simulink model "TractionControl"  (R2024b)
settings: configuration reference "STM32H7_Config" (kept outside this file)
undefined symbols (not defined in the file): Ki1, MMotorMinAllowed, rStraightSlipRatio
libraries: simulink x2
settings Model: DataDictionary=Master_Dictionary.sldd  EnableAccessToBaseWorkspace=off  Creator=torni  LastModifiedBy=William
settings ConfigSetRef: SourceName=STM32H7_Config

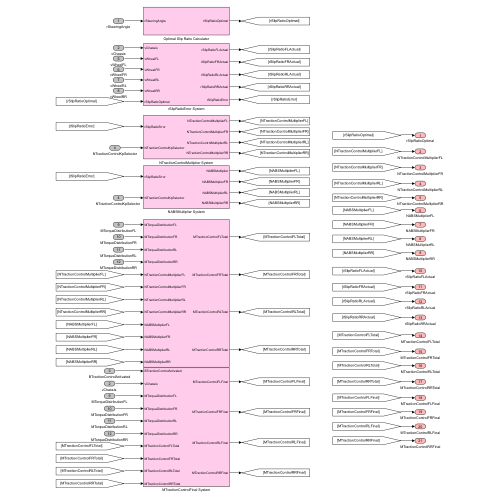
[thumbnail: Simulink's stored preview of the top-level diagram]
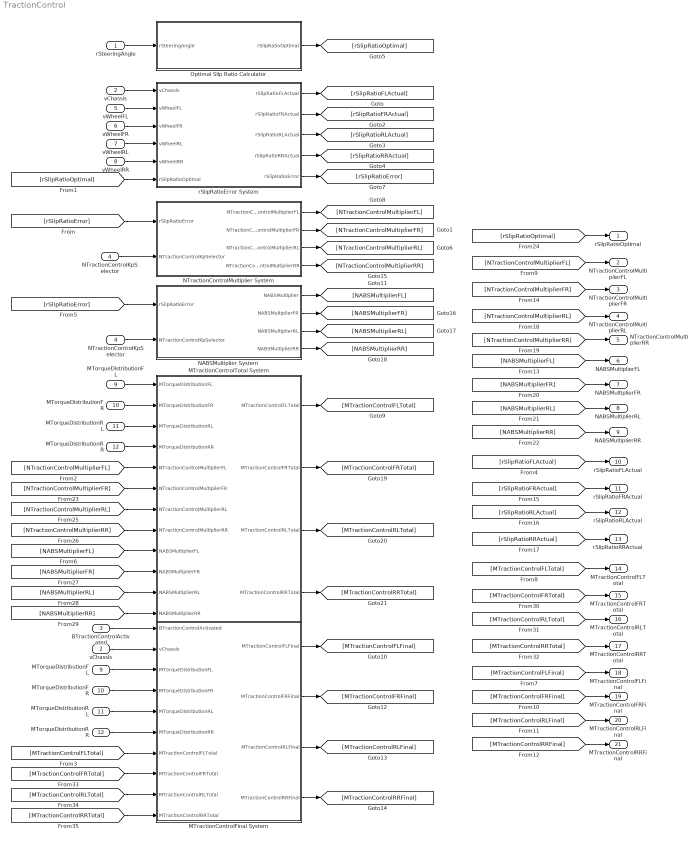
== system TractionControl ==
  rSteeringAngle : Inport  OutDataTypeStr=double
  vChassis : Inport  Port=2  OutDataTypeStr=double
  BTractionControlActivated : Inport  Port=3  OutDataTypeStr=boolean
  NTractionControlKpSelector : Inport  Port=4  OutDataTypeStr=double
  vWheelFL : Inport  Port=5  OutDataTypeStr=double  LockScale=on
  vWheelFR : Inport  Port=6  OutDataTypeStr=double  LockScale=on
  vWheelRL : Inport  Port=7  OutDataTypeStr=double  LockScale=on
  vWheelRR : Inport  Port=8  OutDataTypeStr=double  LockScale=on
  MTorqueDistributionFL : Inport  Port=9  OutDataTypeStr=double
  MTorqueDistributionFR : Inport  Port=10  OutDataTypeStr=double
  MTorqueDistributionRL : Inport  Port=11  OutDataTypeStr=double
  MTorqueDistributionRR : Inport  Port=12  OutDataTypeStr=double
  "MTorqueDistributionFL " : InportShadow  Port=9  OutDataTypeStr=double
  "MTorqueDistributionFR " : InportShadow  Port=10  OutDataTypeStr=double
  "MTorqueDistributionRL " : InportShadow  Port=11  OutDataTypeStr=double
  "MTorqueDistributionRR " : InportShadow  Port=12  OutDataTypeStr=double
  MTractionControlFinal System : Subsystem
  MTractionControlTotal System : Subsystem
  NABSMultiplier System : Subsystem
  "NTractionControlKpSelector " : InportShadow  Port=4  OutDataTypeStr=double
  NTractionControlMultiplier System : Subsystem
  Optimal Slip Ratio Calculator : Subsystem
  rSlipRatioError System : Subsystem
  "vChassis " : InportShadow  Port=2  OutDataTypeStr=double
  rSlipRatioOptimal : Outport  OutDataTypeStr=double  VectorParamsAs1DForOutWhenUnconnected=off
  NTractionControlMultiplierFL : Outport  Port=2  OutDataTypeStr=double  VectorParamsAs1DForOutWhenUnconnected=off
  NTractionControlMultiplierFR : Outport  Port=3  OutDataTypeStr=double  VectorParamsAs1DForOutWhenUnconnected=off
  NTractionControlMultiplierRL : Outport  Port=4  OutDataTypeStr=double  VectorParamsAs1DForOutWhenUnconnected=off
  NTractionControlMultiplierRR : Outport  Port=5  OutDataTypeStr=double  VectorParamsAs1DForOutWhenUnconnected=off
  NABSMultiplierFL : Outport  Port=6  OutDataTypeStr=double  VectorParamsAs1DForOutWhenUnconnected=off
  NABSMultiplierFR : Outport  Port=7  OutDataTypeStr=double  VectorParamsAs1DForOutWhenUnconnected=off
  NABSMultiplierRL : Outport  Port=8  OutDataTypeStr=double  VectorParamsAs1DForOutWhenUnconnected=off
  NABSMultiplierRR : Outport  Port=9  OutDataTypeStr=double  VectorParamsAs1DForOutWhenUnconnected=off
  rSlipRatioFLActual : Outport  Port=10  OutDataTypeStr=double  VectorParamsAs1DForOutWhenUnconnected=off
  rSlipRatioFRActual : Outport  Port=11  OutDataTypeStr=double  VectorParamsAs1DForOutWhenUnconnected=off
  rSlipRatioRLActual : Outport  Port=12  OutDataTypeStr=double  VectorParamsAs1DForOutWhenUnconnected=off
  rSlipRatioRRActual : Outport  Port=13  OutDataTypeStr=double  VectorParamsAs1DForOutWhenUnconnected=off
  MTractionControlFLTotal : Outport  Port=14  OutDataTypeStr=double  VectorParamsAs1DForOutWhenUnconnected=off
  MTractionControlFRTotal : Outport  Port=15  OutDataTypeStr=double  VectorParamsAs1DForOutWhenUnconnected=off
  MTractionControlRLTotal : Outport  Port=16  OutDataTypeStr=double  VectorParamsAs1DForOutWhenUnconnected=off
  MTractionControlRRTotal : Outport  Port=17  OutDataTypeStr=double  VectorParamsAs1DForOutWhenUnconnected=off
  MTractionControlFLFinal : Outport  Port=18  OutDataTypeStr=double  VectorParamsAs1DForOutWhenUnconnected=off
  MTractionControlFRFinal : Outport  Port=19  OutDataTypeStr=double  VectorParamsAs1DForOutWhenUnconnected=off
  MTractionControlRLFinal : Outport  Port=20  OutDataTypeStr=double  VectorParamsAs1DForOutWhenUnconnected=off
  MTractionControlRRFinal : Outport  Port=21  OutDataTypeStr=double  VectorParamsAs1DForOutWhenUnconnected=off
  wires:
  rSteeringAngle/1 -> Optimal Slip Ratio Calculator/1(rSteeringAngle)
  Optimal Slip Ratio Calculator/1(rSlipRatioOptimal) -> [rSlipRatioOptimal]
  [rSlipRatioOptimal] -> rSlipRatioOptimal/1
  MTorqueDistributionFL/1 -> MTractionControlTotal System/1(MTorqueDistributionFL)
  MTorqueDistributionFR/1 -> MTractionControlTotal System/2(MTorqueDistributionFR)
  vWheelRR/1 -> rSlipRatioError System/5(vWheelRR)
  NABSMultiplier System/1(NABSMultiplier) -> [NABSMultiplierFL]
  [rSlipRatioError] -> NTractionControlMultiplier System/1(rSlipRatioError)
  NTractionControlMultiplier System/1(NTractionControlMultiplierFL) -> [NTractionControlMultiplierFL]
  vChassis/1 -> rSlipRatioError System/1(vChassis)
  vWheelFL/1 -> rSlipRatioError System/2(vWheelFL)
  "vChassis "/1 -> MTractionControlFinal System/2(vChassis)
  vWheelFR/1 -> rSlipRatioError System/3(vWheelFR)
  [NTractionControlMultiplierFL] -> NTractionControlMultiplierFL/1
  MTractionControlTotal System/1(MTractionControlFLTotal) -> [MTractionControlFLTotal]
  "MTorqueDistributionFL "/1 -> MTractionControlFinal System/3(MTorqueDistributionFL)
  "NTractionControlKpSelector "/1 -> NABSMultiplier System/2(NTractionControlKpSelector)
  [rSlipRatioError] -> NABSMultiplier System/1(rSlipRatioError)
  "MTorqueDistributionRR "/1 -> MTractionControlFinal System/6(MTorqueDistributionRR)
  BTractionControlActivated/1 -> MTractionControlFinal System/1(BTractionControlActivated)
  "MTorqueDistributionRL "/1 -> MTractionControlFinal System/5(MTorqueDistributionRL)
  [NABSMultiplierFL] -> MTractionControlTotal System/9(NABSMultiplierFL)
  MTorqueDistributionRL/1 -> MTractionControlTotal System/3(MTorqueDistributionRL)
  "MTorqueDistributionFR "/1 -> MTractionControlFinal System/4(MTorqueDistributionFR)
  [NTractionControlMultiplierFL] -> MTractionControlTotal System/5(NTractionControlMultiplierFL)
  MTractionControlFinal System/1(MTractionControlFLFinal) -> [MTractionControlFLFinal]
  rSlipRatioError System/1(rSlipRatioFLActual) -> [rSlipRatioFLActual]
  vWheelRL/1 -> rSlipRatioError System/4(vWheelRL)
  MTractionControlFinal System/3(MTractionControlRLFinal) -> [MTractionControlRLFinal]
  MTractionControlFinal System/4(MTractionControlRRFinal) -> [MTractionControlRRFinal]
  MTractionControlFinal System/2(MTractionControlFRFinal) -> [MTractionControlFRFinal]
  NTractionControlKpSelector/1 -> NTractionControlMultiplier System/2(NTractionControlKpSelector)
  MTorqueDistributionRR/1 -> MTractionControlTotal System/4(MTorqueDistributionRR)
  [rSlipRatioOptimal] -> rSlipRatioError System/6(rSlipRatioOptimal)
  rSlipRatioError System/5(rSlipRatioError) -> [rSlipRatioError]
  rSlipRatioError System/2(rSlipRatioFRActual) -> [rSlipRatioFRActual]
  rSlipRatioError System/3(rSlipRatioRLActual) -> [rSlipRatioRLActual]
  rSlipRatioError System/4(rSlipRatioRRActual) -> [rSlipRatioRRActual]
  NTractionControlMultiplier System/2(NTractionControlMultiplierFR) -> [NTractionControlMultiplierFR]
  NTractionControlMultiplier System/3(NTractionControlMultiplierRL) -> [NTractionControlMultiplierRL]
  NTractionControlMultiplier System/4(NTractionControlMultiplierRR) -> [NTractionControlMultiplierRR]
  [NTractionControlMultiplierFR] -> NTractionControlMultiplierFR/1
  [NTractionControlMultiplierRL] -> NTractionControlMultiplierRL/1
  [NTractionControlMultiplierRR] -> NTractionControlMultiplierRR/1
  [NABSMultiplierFL] -> NABSMultiplierFL/1
  NABSMultiplier System/4(NABSMultiplierRR) -> [NABSMultiplierRR]
  NABSMultiplier System/3(NABSMultiplierRL) -> [NABSMultiplierRL]
  NABSMultiplier System/2(NABSMultiplierFR) -> [NABSMultiplierFR]
  [NTractionControlMultiplierFR] -> MTractionControlTotal System/6(NTractionControlMultiplierFR)
  [NTractionControlMultiplierRL] -> MTractionControlTotal System/7(NTractionControlMultiplierRL)
  [NTractionControlMultiplierRR] -> MTractionControlTotal System/8(NTractionControlMultiplierRR)
  [NABSMultiplierRR] -> NABSMultiplierRR/1
  [NABSMultiplierRL] -> NABSMultiplierRL/1
  [NABSMultiplierFR] -> NABSMultiplierFR/1
  [NABSMultiplierFR] -> MTractionControlTotal System/10(NABSMultiplierFR)
  [NABSMultiplierRL] -> MTractionControlTotal System/11(NABSMultiplierRL)
  [NABSMultiplierRR] -> MTractionControlTotal System/12(NABSMultiplierRR)
  [rSlipRatioRRActual] -> rSlipRatioRRActual/1
  [rSlipRatioFLActual] -> rSlipRatioFLActual/1
  [rSlipRatioFRActual] -> rSlipRatioFRActual/1
  [rSlipRatioRLActual] -> rSlipRatioRLActual/1
  MTractionControlTotal System/2(MTractionControlFRTotal) -> [MTractionControlFRTotal]
  MTractionControlTotal System/3(MTractionControlRLTotal) -> [MTractionControlRLTotal]
  MTractionControlTotal System/4(MTractionControlRRTotal) -> [MTractionControlRRTotal]
  [MTractionControlFLTotal] -> MTractionControlFLTotal/1
  [MTractionControlFRTotal] -> MTractionControlFRTotal/1
  [MTractionControlRLTotal] -> MTractionControlRLTotal/1
  [MTractionControlRRTotal] -> MTractionControlRRTotal/1
  [MTractionControlFLFinal] -> MTractionControlFLFinal/1
  [MTractionControlRRFinal] -> MTractionControlRRFinal/1
  [MTractionControlFRFinal] -> MTractionControlFRFinal/1
  [MTractionControlRLFinal] -> MTractionControlRLFinal/1
  [MTractionControlFLTotal] -> MTractionControlFinal System/7(MTractionControlFLTotal)
  [MTractionControlFRTotal] -> MTractionControlFinal System/8(MTractionControlFRTotal)
  [MTractionControlRLTotal] -> MTractionControlFinal System/9(MTractionControlRLTotal)
  [MTractionControlRRTotal] -> MTractionControlFinal System/10(MTractionControlRRTotal)

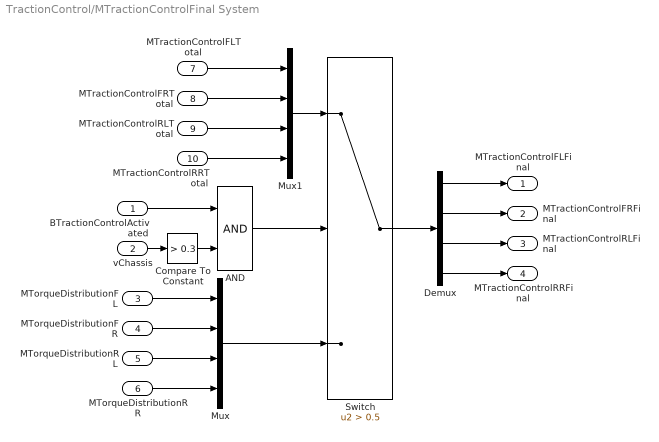
== system TractionControl/MTractionControlFinal System ==
  BTractionControlActivated : Inport  OutDataTypeStr=boolean
  vChassis : Inport  Port=2  OutDataTypeStr=double
  MTorqueDistributionFL : Inport  Port=3  OutDataTypeStr=double
  MTorqueDistributionFR : Inport  Port=4  OutDataTypeStr=double
  MTorqueDistributionRL : Inport  Port=5  OutDataTypeStr=double
  MTorqueDistributionRR : Inport  Port=6  OutDataTypeStr=double
  MTractionControlFLTotal : Inport  Port=7  OutDataTypeStr=double
  MTractionControlFRTotal : Inport  Port=8  OutDataTypeStr=double
  MTractionControlRLTotal : Inport  Port=9  OutDataTypeStr=double
  MTractionControlRRTotal : Inport  Port=10  OutDataTypeStr=double
  AND : Logic  AllPortsSameDT=off  OutDataTypeStr=boolean
  Compare To Constant : simulink/Logic and Bit Operations/Compare To Constant  relop=>  const=0.3  OutDataTypeStr=boolean
  Demux : Demux
  Mux : Mux
  Mux1 : Mux
  Switch : Switch  Criteria=u2 > Threshold  Threshold=0.5  SaturateOnIntegerOverflow=off  InputSameDT=off
  MTractionControlFLFinal : Outport  OutDataTypeStr=double  VectorParamsAs1DForOutWhenUnconnected=off
  MTractionControlFRFinal : Outport  Port=2  OutDataTypeStr=double  VectorParamsAs1DForOutWhenUnconnected=off
  MTractionControlRLFinal : Outport  Port=3  OutDataTypeStr=double  VectorParamsAs1DForOutWhenUnconnected=off
  MTractionControlRRFinal : Outport  Port=4  OutDataTypeStr=double  VectorParamsAs1DForOutWhenUnconnected=off
  wires:
  Mux/1 -> Switch/3
  BTractionControlActivated/1 -> AND/1
  vChassis/1 -> Compare To Constant/1
  AND/1 -> Switch/2
  Compare To Constant/1 -> AND/2
  MTorqueDistributionRL/1 -> Mux/3
  MTorqueDistributionFR/1 -> Mux/2
  MTorqueDistributionRR/1 -> Mux/4
  MTorqueDistributionFL/1 -> Mux/1
  Demux/4 -> MTractionControlRRFinal/1
  Switch/1 -> Demux/1
  Demux/1 -> MTractionControlFLFinal/1
  Demux/2 -> MTractionControlFRFinal/1
  Demux/3 -> MTractionControlRLFinal/1
  Mux1/1 -> Switch/1
  MTractionControlRRTotal/1 -> Mux1/4
  MTractionControlRLTotal/1 -> Mux1/3
  MTractionControlFRTotal/1 -> Mux1/2
  MTractionControlFLTotal/1 -> Mux1/1

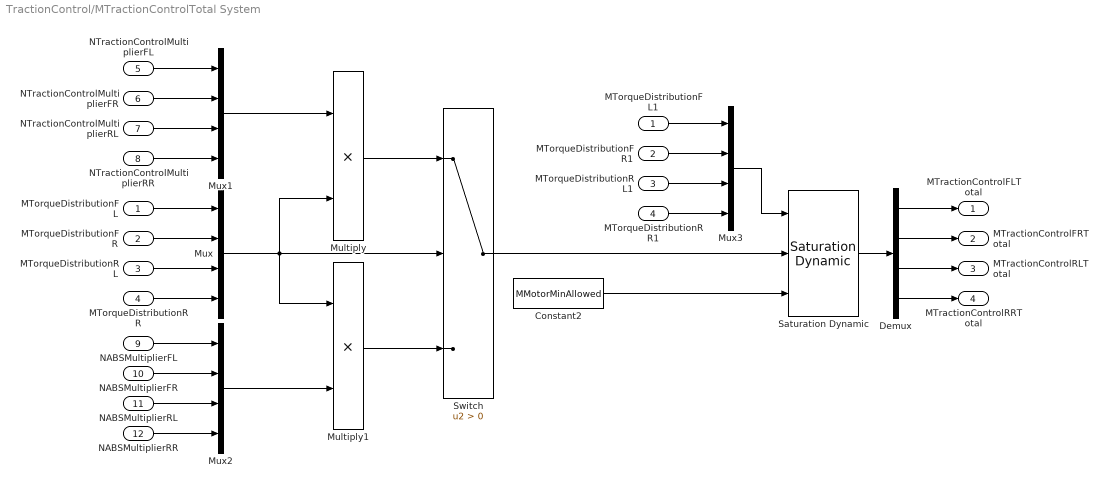
== system TractionControl/MTractionControlTotal System ==
  MTorqueDistributionFL : Inport  OutDataTypeStr=double
  MTorqueDistributionFR : Inport  Port=2  OutDataTypeStr=double
  MTorqueDistributionRL : Inport  Port=3  OutDataTypeStr=double
  MTorqueDistributionRR : Inport  Port=4  OutDataTypeStr=double
  NTractionControlMultiplierFL : Inport  Port=5  OutDataTypeStr=double
  NTractionControlMultiplierFR : Inport  Port=6  OutDataTypeStr=double
  NTractionControlMultiplierRL : Inport  Port=7  OutDataTypeStr=double
  NTractionControlMultiplierRR : Inport  Port=8  OutDataTypeStr=double
  NABSMultiplierFL : Inport  Port=9  OutDataTypeStr=double
  NABSMultiplierFR : Inport  Port=10  OutDataTypeStr=double
  NABSMultiplierRL : Inport  Port=11  OutDataTypeStr=double
  NABSMultiplierRR : Inport  Port=12  OutDataTypeStr=double
  Constant2 : Constant  Value=MMotorMinAllowed
  Demux : Demux
  MTorqueDistributionFL1 : InportShadow  OutDataTypeStr=double
  MTorqueDistributionFR1 : InportShadow  Port=2  OutDataTypeStr=double
  MTorqueDistributionRL1 : InportShadow  Port=3  OutDataTypeStr=double
  MTorqueDistributionRR1 : InportShadow  Port=4  OutDataTypeStr=double
  Multiply : Product
  Multiply1 : Product
  Mux{,1..3} (4 alike) : Mux
  Saturation Dynamic : simulink/Discontinuities/Saturation Dynamic  OutMin=[]  OutMax=[]  OutDataTypeStr=Inherit: Same as second input  OutDataType=fixdt(1, 16)  OutScaling=2^-10  DoSatur=off
  Switch : Switch  Criteria=u2 > Threshold  SaturateOnIntegerOverflow=off  InputSameDT=off
  MTractionControlFLTotal : Outport  OutDataTypeStr=double  VectorParamsAs1DForOutWhenUnconnected=off
  MTractionControlFRTotal : Outport  Port=2  OutDataTypeStr=double  VectorParamsAs1DForOutWhenUnconnected=off
  MTractionControlRLTotal : Outport  Port=3  OutDataTypeStr=double  VectorParamsAs1DForOutWhenUnconnected=off
  MTractionControlRRTotal : Outport  Port=4  OutDataTypeStr=double  VectorParamsAs1DForOutWhenUnconnected=off
  wires:
  Multiply/1 -> Switch/1
  Constant2/1 -> Saturation Dynamic/3
  Switch/1 -> Saturation Dynamic/2
  Multiply1/1 -> Switch/3
  Mux/1 -> Multiply1/1, Switch/2, Multiply/2
  MTorqueDistributionFL/1 -> Mux/1
  MTorqueDistributionFR/1 -> Mux/2
  MTorqueDistributionRL/1 -> Mux/3
  MTorqueDistributionRR/1 -> Mux/4
  Mux1/1 -> Multiply/1
  NTractionControlMultiplierRR/1 -> Mux1/4
  NTractionControlMultiplierRL/1 -> Mux1/3
  NTractionControlMultiplierFR/1 -> Mux1/2
  NTractionControlMultiplierFL/1 -> Mux1/1
  NABSMultiplierFL/1 -> Mux2/1
  NABSMultiplierRL/1 -> Mux2/3
  NABSMultiplierRR/1 -> Mux2/4
  NABSMultiplierFR/1 -> Mux2/2
  Mux2/1 -> Multiply1/2
  Saturation Dynamic/1 -> Demux/1
  Demux/1 -> MTractionControlFLTotal/1
  Demux/2 -> MTractionControlFRTotal/1
  Demux/3 -> MTractionControlRLTotal/1
  Demux/4 -> MTractionControlRRTotal/1
  Mux3/1 -> Saturation Dynamic/1
  MTorqueDistributionFL1/1 -> Mux3/1
  MTorqueDistributionRL1/1 -> Mux3/3
  MTorqueDistributionFR1/1 -> Mux3/2
  MTorqueDistributionRR1/1 -> Mux3/4

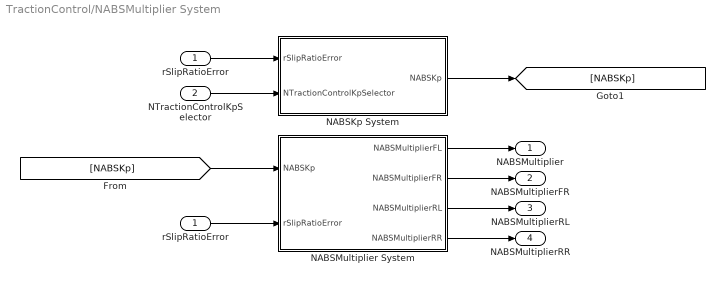
== system TractionControl/NABSMultiplier System ==
  rSlipRatioError : Inport  OutDataTypeStr=double
  NTractionControlKpSelector : Inport  Port=2  OutDataTypeStr=double
  NABSKp System : Subsystem
  NABSMultiplier System : Subsystem
  "rSlipRatioError " : InportShadow  OutDataTypeStr=double
  NABSMultiplier : Outport  OutDataTypeStr=double  VectorParamsAs1DForOutWhenUnconnected=off
  NABSMultiplierFR : Outport  Port=2  OutDataTypeStr=double  VectorParamsAs1DForOutWhenUnconnected=off
  NABSMultiplierRL : Outport  Port=3  OutDataTypeStr=double  VectorParamsAs1DForOutWhenUnconnected=off
  NABSMultiplierRR : Outport  Port=4  OutDataTypeStr=double  VectorParamsAs1DForOutWhenUnconnected=off
  wires:
  NTractionControlKpSelector/1 -> NABSKp System/2(NTractionControlKpSelector)
  rSlipRatioError/1 -> NABSKp System/1(rSlipRatioError)
  NABSKp System/1(NABSKp) -> [NABSKp]
  "rSlipRatioError "/1 -> NABSMultiplier System/2(rSlipRatioError)
  [NABSKp] -> NABSMultiplier System/1(NABSKp)
  NABSMultiplier System/1(NABSMultiplierFL) -> NABSMultiplier/1
  NABSMultiplier System/2(NABSMultiplierFR) -> NABSMultiplierFR/1
  NABSMultiplier System/3(NABSMultiplierRL) -> NABSMultiplierRL/1
  NABSMultiplier System/4(NABSMultiplierRR) -> NABSMultiplierRR/1

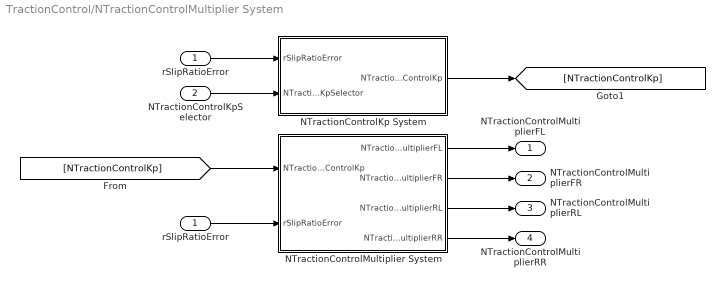
== system TractionControl/NTractionControlMultiplier System ==
  rSlipRatioError : Inport  OutDataTypeStr=double
  NTractionControlKpSelector : Inport  Port=2  OutDataTypeStr=double  LockScale=on
  NTractionControlKp System : Subsystem
  NTractionControlMultiplier System : Subsystem
  "rSlipRatioError " : InportShadow  OutDataTypeStr=double
  NTractionControlMultiplierFL : Outport  OutDataTypeStr=double  VectorParamsAs1DForOutWhenUnconnected=off
  NTractionControlMultiplierFR : Outport  Port=2  OutDataTypeStr=double  VectorParamsAs1DForOutWhenUnconnected=off
  NTractionControlMultiplierRL : Outport  Port=3  OutDataTypeStr=double  VectorParamsAs1DForOutWhenUnconnected=off
  NTractionControlMultiplierRR : Outport  Port=4  OutDataTypeStr=double  VectorParamsAs1DForOutWhenUnconnected=off
  wires:
  [NTractionControlKp] -> NTractionControlMultiplier System/1(NTractionControlKp)
  "rSlipRatioError "/1 -> NTractionControlMultiplier System/2(rSlipRatioError)
  NTractionControlKp System/1(NTractionControlKp) -> [NTractionControlKp]
  rSlipRatioError/1 -> NTractionControlKp System/1(rSlipRatioError)
  NTractionControlKpSelector/1 -> NTractionControlKp System/2(NTractionControlKpSelector)
  NTractionControlMultiplier System/1(NTractionControlMultiplierFL) -> NTractionControlMultiplierFL/1
  NTractionControlMultiplier System/2(NTractionControlMultiplierFR) -> NTractionControlMultiplierFR/1
  NTractionControlMultiplier System/3(NTractionControlMultiplierRL) -> NTractionControlMultiplierRL/1
  NTractionControlMultiplier System/4(NTractionControlMultiplierRR) -> NTractionControlMultiplierRR/1

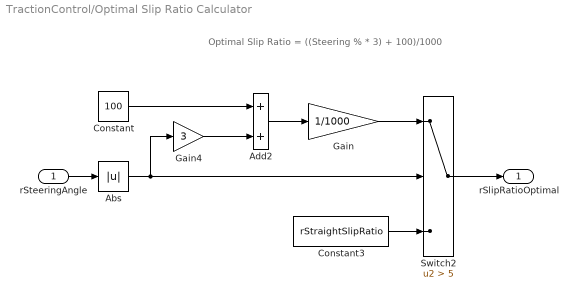
== system TractionControl/Optimal Slip Ratio Calculator ==
  note: Optimal Slip Ratio = ((Steering % * 3) + 100)/1000
  rSteeringAngle : Inport  OutDataTypeStr=double
  Abs : Abs  SaturateOnIntegerOverflow=off
  Add2 : Sum
  Constant : Constant  Value=100
  Constant3 : Constant  Value=rStraightSlipRatio
  Gain : Gain  Gain=1/1000
  Gain4 : Gain  Gain=3
  Switch2 : Switch  Criteria=u2 > Threshold  Threshold=5  SaturateOnIntegerOverflow=off  InputSameDT=off
  rSlipRatioOptimal : Outport  OutDataTypeStr=double  VectorParamsAs1DForOutWhenUnconnected=off
  wires:
  Add2/1 -> Gain/1
  Constant/1 -> Add2/1
  rSteeringAngle/1 -> Abs/1
  Gain/1 -> Switch2/1
  Constant3/1 -> Switch2/3
  Gain4/1 -> Add2/2
  Switch2/1 -> rSlipRatioOptimal/1
  Abs/1 -> Gain4/1, Switch2/2

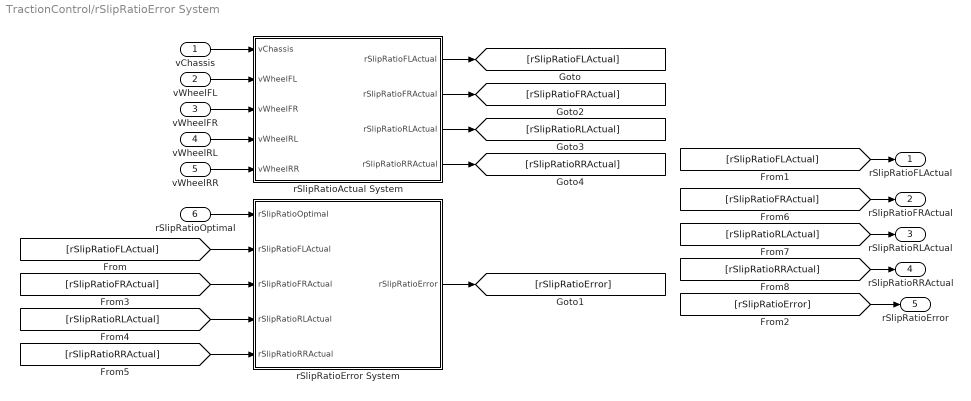
== system TractionControl/rSlipRatioError System ==
  vChassis : Inport  OutDataTypeStr=double
  vWheelFL : Inport  Port=2  OutDataTypeStr=double  LockScale=on
  vWheelFR : Inport  Port=3  OutDataTypeStr=double  LockScale=on
  vWheelRL : Inport  Port=4  OutDataTypeStr=double  LockScale=on
  vWheelRR : Inport  Port=5  OutDataTypeStr=double  LockScale=on
  rSlipRatioOptimal : Inport  Port=6  OutDataTypeStr=double
  rSlipRatioActual System : Subsystem
  rSlipRatioError System : Subsystem
  rSlipRatioFLActual : Outport  OutDataTypeStr=double  VectorParamsAs1DForOutWhenUnconnected=off
  rSlipRatioFRActual : Outport  Port=2  OutDataTypeStr=double  VectorParamsAs1DForOutWhenUnconnected=off
  rSlipRatioRLActual : Outport  Port=3  OutDataTypeStr=double  VectorParamsAs1DForOutWhenUnconnected=off
  rSlipRatioRRActual : Outport  Port=4  OutDataTypeStr=double  VectorParamsAs1DForOutWhenUnconnected=off
  rSlipRatioError : Outport  Port=5  OutDataTypeStr=double  VectorParamsAs1DForOutWhenUnconnected=off
  wires:
  rSlipRatioError System/1(rSlipRatioError) -> [rSlipRatioError]
  [rSlipRatioFLActual] -> rSlipRatioError System/2(rSlipRatioFLActual)
  rSlipRatioOptimal/1 -> rSlipRatioError System/1(rSlipRatioOptimal)
  [rSlipRatioFLActual] -> rSlipRatioFLActual/1
  [rSlipRatioError] -> rSlipRatioError/1
  rSlipRatioActual System/1(rSlipRatioFLActual) -> [rSlipRatioFLActual]
  vChassis/1 -> rSlipRatioActual System/1(vChassis)
  vWheelFL/1 -> rSlipRatioActual System/2(vWheelFL)
  vWheelFR/1 -> rSlipRatioActual System/3(vWheelFR)
  vWheelRL/1 -> rSlipRatioActual System/4(vWheelRL)
  vWheelRR/1 -> rSlipRatioActual System/5(vWheelRR)
  rSlipRatioActual System/2(rSlipRatioFRActual) -> [rSlipRatioFRActual]
  rSlipRatioActual System/3(rSlipRatioRLActual) -> [rSlipRatioRLActual]
  rSlipRatioActual System/4(rSlipRatioRRActual) -> [rSlipRatioRRActual]
  [rSlipRatioFRActual] -> rSlipRatioError System/3(rSlipRatioFRActual)
  [rSlipRatioRLActual] -> rSlipRatioError System/4(rSlipRatioRLActual)
  [rSlipRatioRRActual] -> rSlipRatioError System/5(rSlipRatioRRActual)
  [rSlipRatioFRActual] -> rSlipRatioFRActual/1
  [rSlipRatioRLActual] -> rSlipRatioRLActual/1
  [rSlipRatioRRActual] -> rSlipRatioRRActual/1

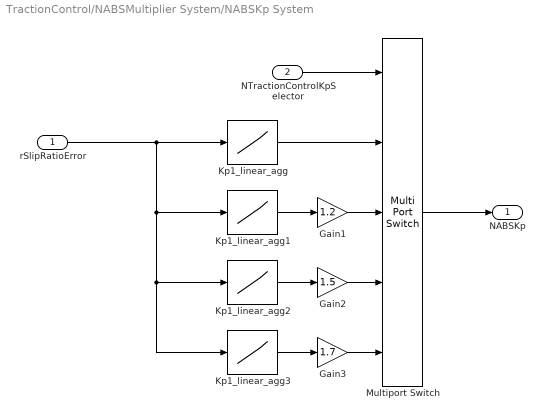
== system TractionControl/NABSMultiplier System/NABSKp System ==
  rSlipRatioError : Inport  OutDataTypeStr=double
  NTractionControlKpSelector : Inport  Port=2  OutDataTypeStr=double
  Gain1 : Gain  Gain=1.2
  Gain2 : Gain  Gain=1.5
  Gain3 : Gain  Gain=1.7
  Kp1_linear_agg : Lookup_n-D  NumberOfTableDimensions=1  BreakpointsForDimension1=|  BreakpointsForDimension2=Ki1  Table=|  InternalRulePriority=Speed  RndMeth=Simplest
      BreakpointsForDimension1=|
      | [0.10
      | 0.11
      | 0.12
      | 0.13
      | 0.14
      | 0.15
      | 0.16
      | 0.17
      | 0.18
      | 0.19
      | 0.20
      | 0.21
      | 0.22
      | 0.23
      | 0.24
      | 0.25
      | 0.26
      | 0.27
      | 0.28
      | 0.29
      | 0.30
      | 0.31
      | 0.32
      | 0.33
      | 0.34
      | 0.35
      | 0.36
      | 0.37
      | 0.38
      | 0.39
      | 0.40
      | 0.41
      | 0.42
      | 0.43
      | 0.44
      | 0.45
      | 0.46
      | 0.47
      | 0.48
      | 0.49
      | 0.50
      | ]
      Table=|
      | [0.1
      | 0.1175
      | 0.135
      | 0.1525
      | 0.17
      | 0.1875
      | 0.205
      | 0.2225
      | 0.24
      | 0.2575
      | 0.275
      | 0.2925
      | 0.31
      | 0.3275
      | 0.345
      | 0.3625
      | 0.38
      | 0.3975
      | 0.415
      | 0.4325
      | 0.45
      | 0.4675
      | 0.485
      | 0.5025
      | 0.52
      | 0.5375
      | 0.555
      | 0.5725
      | 0.59
      | 0.6075
      | 0.625
      | 0.6425
      | 0.66
      | 0.6775
      | 0.695
      | 0.7125
      | 0.73
      | 0.7475
      | 0.765
      | 0.7825
      | 0.8
      | ]
  Kp1_linear_agg1 : Lookup_n-D  NumberOfTableDimensions=1  BreakpointsForDimension1=|  BreakpointsForDimension2=Ki1  Table=|  InternalRulePriority=Speed  RndMeth=Simplest
      BreakpointsForDimension1=|
      | [0.10
      | 0.11
      | 0.12
      | 0.13
      | 0.14
      | 0.15
      | 0.16
      | 0.17
      | 0.18
      | 0.19
      | 0.20
      | 0.21
      | 0.22
      | 0.23
      | 0.24
      | 0.25
      | 0.26
      | 0.27
      | 0.28
      | 0.29
      | 0.30
      | 0.31
      | 0.32
      | 0.33
      | 0.34
      | 0.35
      | 0.36
      | 0.37
      | 0.38
      | 0.39
      | 0.40
      | 0.41
      | 0.42
      | 0.43
      | 0.44
      | 0.45
      | 0.46
      | 0.47
      | 0.48
      | 0.49
      | 0.50
      | ]
      Table=|
      | [0.1
      | 0.1175
      | 0.135
      | 0.1525
      | 0.17
      | 0.1875
      | 0.205
      | 0.2225
      | 0.24
      | 0.2575
      | 0.275
      | 0.2925
      | 0.31
      | 0.3275
      | 0.345
      | 0.3625
      | 0.38
      | 0.3975
      | 0.415
      | 0.4325
      | 0.45
      | 0.4675
      | 0.485
      | 0.5025
      | 0.52
      | 0.5375
      | 0.555
      | 0.5725
      | 0.59
      | 0.6075
      | 0.625
      | 0.6425
      | 0.66
      | 0.6775
      | 0.695
      | 0.7125
      | 0.73
      | 0.7475
      | 0.765
      | 0.7825
      | 0.8
      | ]
  Kp1_linear_agg2 : Lookup_n-D  NumberOfTableDimensions=1  BreakpointsForDimension1=|  BreakpointsForDimension2=Ki1  Table=|  InternalRulePriority=Speed  RndMeth=Simplest
      BreakpointsForDimension1=|
      | [0.10
      | 0.11
      | 0.12
      | 0.13
      | 0.14
      | 0.15
      | 0.16
      | 0.17
      | 0.18
      | 0.19
      | 0.20
      | 0.21
      | 0.22
      | 0.23
      | 0.24
      | 0.25
      | 0.26
      | 0.27
      | 0.28
      | 0.29
      | 0.30
      | 0.31
      | 0.32
      | 0.33
      | 0.34
      | 0.35
      | 0.36
      | 0.37
      | 0.38
      | 0.39
      | 0.40
      | 0.41
      | 0.42
      | 0.43
      | 0.44
      | 0.45
      | 0.46
      | 0.47
      | 0.48
      | 0.49
      | 0.50
      | ]
      Table=|
      | [0.1
      | 0.1175
      | 0.135
      | 0.1525
      | 0.17
      | 0.1875
      | 0.205
      | 0.2225
      | 0.24
      | 0.2575
      | 0.275
      | 0.2925
      | 0.31
      | 0.3275
      | 0.345
      | 0.3625
      | 0.38
      | 0.3975
      | 0.415
      | 0.4325
      | 0.45
      | 0.4675
      | 0.485
      | 0.5025
      | 0.52
      | 0.5375
      | 0.555
      | 0.5725
      | 0.59
      | 0.6075
      | 0.625
      | 0.6425
      | 0.66
      | 0.6775
      | 0.695
      | 0.7125
      | 0.73
      | 0.7475
      | 0.765
      | 0.7825
      | 0.8
      | ]
  Kp1_linear_agg3 : Lookup_n-D  NumberOfTableDimensions=1  BreakpointsForDimension1=|  BreakpointsForDimension2=Ki1  Table=|  InternalRulePriority=Speed  RndMeth=Simplest
      BreakpointsForDimension1=|
      | [0.10
      | 0.11
      | 0.12
      | 0.13
      | 0.14
      | 0.15
      | 0.16
      | 0.17
      | 0.18
      | 0.19
      | 0.20
      | 0.21
      | 0.22
      | 0.23
      | 0.24
      | 0.25
      | 0.26
      | 0.27
      | 0.28
      | 0.29
      | 0.30
      | 0.31
      | 0.32
      | 0.33
      | 0.34
      | 0.35
      | 0.36
      | 0.37
      | 0.38
      | 0.39
      | 0.40
      | 0.41
      | 0.42
      | 0.43
      | 0.44
      | 0.45
      | 0.46
      | 0.47
      | 0.48
      | 0.49
      | 0.50
      | ]
      Table=|
      | [0.1
      | 0.1175
      | 0.135
      | 0.1525
      | 0.17
      | 0.1875
      | 0.205
      | 0.2225
      | 0.24
      | 0.2575
      | 0.275
      | 0.2925
      | 0.31
      | 0.3275
      | 0.345
      | 0.3625
      | 0.38
      | 0.3975
      | 0.415
      | 0.4325
      | 0.45
      | 0.4675
      | 0.485
      | 0.5025
      | 0.52
      | 0.5375
      | 0.555
      | 0.5725
      | 0.59
      | 0.6075
      | 0.625
      | 0.6425
      | 0.66
      | 0.6775
      | 0.695
      | 0.7125
      | 0.73
      | 0.7475
      | 0.765
      | 0.7825
      | 0.8
      | ]
  Multiport Switch : MultiPortSwitch  Inputs=4  SaturateOnIntegerOverflow=off  InputSameDT=off
  NABSKp : Outport  OutDataTypeStr=double  VectorParamsAs1DForOutWhenUnconnected=off
  wires:
  rSlipRatioError/1 -> Kp1_linear_agg3/1, Kp1_linear_agg2/1, Kp1_linear_agg1/1, Kp1_linear_agg/1
  NTractionControlKpSelector/1 -> Multiport Switch/1
  Kp1_linear_agg/1 -> Multiport Switch/2
  Kp1_linear_agg3/1 -> Gain3/1
  Kp1_linear_agg2/1 -> Gain2/1
  Kp1_linear_agg1/1 -> Gain1/1
  Multiport Switch/1 -> NABSKp/1
  Gain1/1 -> Multiport Switch/3
  Gain2/1 -> Multiport Switch/4
  Gain3/1 -> Multiport Switch/5

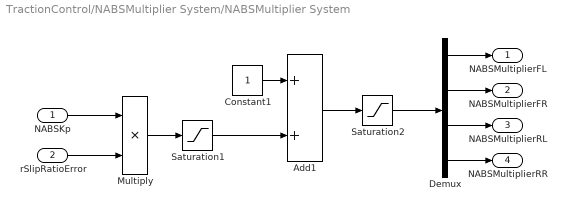
== system TractionControl/NABSMultiplier System/NABSMultiplier System ==
  NABSKp : Inport  OutDataTypeStr=double
  rSlipRatioError : Inport  Port=2  OutDataTypeStr=double
  Add1 : Sum
  Constant1 : Constant
  Demux : Demux
  Multiply : Product
  Saturation1 : Saturate  UpperLimit=0  LowerLimit=-0.8
  Saturation2 : Saturate  UpperLimit=1  LowerLimit=0.2
  NABSMultiplierFL : Outport  OutDataTypeStr=double  VectorParamsAs1DForOutWhenUnconnected=off
  NABSMultiplierFR : Outport  Port=2  OutDataTypeStr=double  VectorParamsAs1DForOutWhenUnconnected=off
  NABSMultiplierRL : Outport  Port=3  OutDataTypeStr=double  VectorParamsAs1DForOutWhenUnconnected=off
  NABSMultiplierRR : Outport  Port=4  OutDataTypeStr=double  VectorParamsAs1DForOutWhenUnconnected=off
  wires:
  Multiply/1 -> Saturation1/1
  NABSKp/1 -> Multiply/1
  rSlipRatioError/1 -> Multiply/2
  Constant1/1 -> Add1/1
  Add1/1 -> Saturation2/1
  Saturation1/1 -> Add1/2
  Demux/4 -> NABSMultiplierRR/1
  Demux/3 -> NABSMultiplierRL/1
  Demux/2 -> NABSMultiplierFR/1
  Demux/1 -> NABSMultiplierFL/1
  Saturation2/1 -> Demux/1

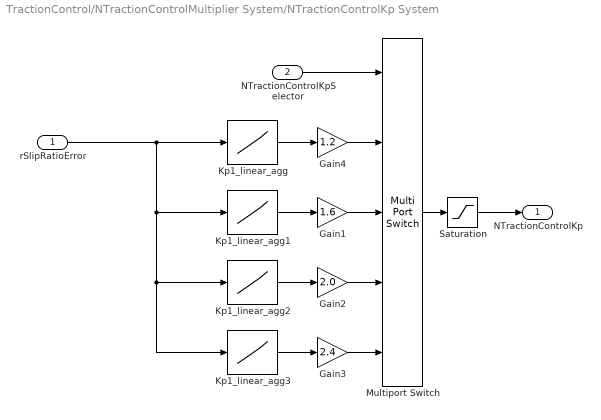
== system TractionControl/NTractionControlMultiplier System/NTractionControlKp System ==
  rSlipRatioError : Inport  OutDataTypeStr=double
  NTractionControlKpSelector : Inport  Port=2  OutDataTypeStr=double
  Gain1 : Gain  Gain=1.6
  Gain2 : Gain  Gain=2.0
  Gain3 : Gain  Gain=2.4
  Gain4 : Gain  Gain=1.2
  Kp1_linear_agg : Lookup_n-D  NumberOfTableDimensions=1  BreakpointsForDimension1=|  BreakpointsForDimension2=Ki1  Table=|  InternalRulePriority=Speed  RndMeth=Simplest
      BreakpointsForDimension1=|
      | [0.10
      | 0.11
      | 0.12
      | 0.13
      | 0.14
      | 0.15
      | 0.16
      | 0.17
      | 0.18
      | 0.19
      | 0.20
      | 0.21
      | 0.22
      | 0.23
      | 0.24
      | 0.25
      | 0.26
      | 0.27
      | 0.28
      | 0.29
      | 0.30
      | 0.31
      | 0.32
      | 0.33
      | 0.34
      | 0.35
      | 0.36
      | 0.37
      | 0.38
      | 0.39
      | 0.40
      | 0.41
      | 0.42
      | 0.43
      | 0.44
      | 0.45
      | 0.46
      | 0.47
      | 0.48
      | 0.49
      | 0.50
      | ]
      Table=|
      | [0.1
      | 0.1175
      | 0.135
      | 0.1525
      | 0.17
      | 0.1875
      | 0.205
      | 0.2225
      | 0.24
      | 0.2575
      | 0.275
      | 0.2925
      | 0.31
      | 0.3275
      | 0.345
      | 0.3625
      | 0.38
      | 0.3975
      | 0.415
      | 0.4325
      | 0.45
      | 0.4675
      | 0.485
      | 0.5025
      | 0.52
      | 0.5375
      | 0.555
      | 0.5725
      | 0.59
      | 0.6075
      | 0.625
      | 0.6425
      | 0.66
      | 0.6775
      | 0.695
      | 0.7125
      | 0.73
      | 0.7475
      | 0.765
      | 0.7825
      | 0.8
      | ]
  Kp1_linear_agg1 : Lookup_n-D  NumberOfTableDimensions=1  BreakpointsForDimension1=|  BreakpointsForDimension2=Ki1  Table=|  InternalRulePriority=Speed  RndMeth=Simplest
      BreakpointsForDimension1=|
      | [0.10
      | 0.11
      | 0.12
      | 0.13
      | 0.14
      | 0.15
      | 0.16
      | 0.17
      | 0.18
      | 0.19
      | 0.20
      | 0.21
      | 0.22
      | 0.23
      | 0.24
      | 0.25
      | 0.26
      | 0.27
      | 0.28
      | 0.29
      | 0.30
      | 0.31
      | 0.32
      | 0.33
      | 0.34
      | 0.35
      | 0.36
      | 0.37
      | 0.38
      | 0.39
      | 0.40
      | 0.41
      | 0.42
      | 0.43
      | 0.44
      | 0.45
      | 0.46
      | 0.47
      | 0.48
      | 0.49
      | 0.50
      | ]
      Table=|
      | [0.1
      | 0.1175
      | 0.135
      | 0.1525
      | 0.17
      | 0.1875
      | 0.205
      | 0.2225
      | 0.24
      | 0.2575
      | 0.275
      | 0.2925
      | 0.31
      | 0.3275
      | 0.345
      | 0.3625
      | 0.38
      | 0.3975
      | 0.415
      | 0.4325
      | 0.45
      | 0.4675
      | 0.485
      | 0.5025
      | 0.52
      | 0.5375
      | 0.555
      | 0.5725
      | 0.59
      | 0.6075
      | 0.625
      | 0.6425
      | 0.66
      | 0.6775
      | 0.695
      | 0.7125
      | 0.73
      | 0.7475
      | 0.765
      | 0.7825
      | 0.8
      | ]
  Kp1_linear_agg2 : Lookup_n-D  NumberOfTableDimensions=1  BreakpointsForDimension1=|  BreakpointsForDimension2=Ki1  Table=|  InternalRulePriority=Speed  RndMeth=Simplest
      BreakpointsForDimension1=|
      | [0.10
      | 0.11
      | 0.12
      | 0.13
      | 0.14
      | 0.15
      | 0.16
      | 0.17
      | 0.18
      | 0.19
      | 0.20
      | 0.21
      | 0.22
      | 0.23
      | 0.24
      | 0.25
      | 0.26
      | 0.27
      | 0.28
      | 0.29
      | 0.30
      | 0.31
      | 0.32
      | 0.33
      | 0.34
      | 0.35
      | 0.36
      | 0.37
      | 0.38
      | 0.39
      | 0.40
      | 0.41
      | 0.42
      | 0.43
      | 0.44
      | 0.45
      | 0.46
      | 0.47
      | 0.48
      | 0.49
      | 0.50
      | ]
      Table=|
      | [0.1
      | 0.1175
      | 0.135
      | 0.1525
      | 0.17
      | 0.1875
      | 0.205
      | 0.2225
      | 0.24
      | 0.2575
      | 0.275
      | 0.2925
      | 0.31
      | 0.3275
      | 0.345
      | 0.3625
      | 0.38
      | 0.3975
      | 0.415
      | 0.4325
      | 0.45
      | 0.4675
      | 0.485
      | 0.5025
      | 0.52
      | 0.5375
      | 0.555
      | 0.5725
      | 0.59
      | 0.6075
      | 0.625
      | 0.6425
      | 0.66
      | 0.6775
      | 0.695
      | 0.7125
      | 0.73
      | 0.7475
      | 0.765
      | 0.7825
      | 0.8
      | ]
  Kp1_linear_agg3 : Lookup_n-D  NumberOfTableDimensions=1  BreakpointsForDimension1=|  BreakpointsForDimension2=Ki1  Table=|  InternalRulePriority=Speed  RndMeth=Simplest
      BreakpointsForDimension1=|
      | [0.10
      | 0.11
      | 0.12
      | 0.13
      | 0.14
      | 0.15
      | 0.16
      | 0.17
      | 0.18
      | 0.19
      | 0.20
      | 0.21
      | 0.22
      | 0.23
      | 0.24
      | 0.25
      | 0.26
      | 0.27
      | 0.28
      | 0.29
      | 0.30
      | 0.31
      | 0.32
      | 0.33
      | 0.34
      | 0.35
      | 0.36
      | 0.37
      | 0.38
      | 0.39
      | 0.40
      | 0.41
      | 0.42
      | 0.43
      | 0.44
      | 0.45
      | 0.46
      | 0.47
      | 0.48
      | 0.49
      | 0.50
      | ]
      Table=|
      | [0.1
      | 0.1175
      | 0.135
      | 0.1525
      | 0.17
      | 0.1875
      | 0.205
      | 0.2225
      | 0.24
      | 0.2575
      | 0.275
      | 0.2925
      | 0.31
      | 0.3275
      | 0.345
      | 0.3625
      | 0.38
      | 0.3975
      | 0.415
      | 0.4325
      | 0.45
      | 0.4675
      | 0.485
      | 0.5025
      | 0.52
      | 0.5375
      | 0.555
      | 0.5725
      | 0.59
      | 0.6075
      | 0.625
      | 0.6425
      | 0.66
      | 0.6775
      | 0.695
      | 0.7125
      | 0.73
      | 0.7475
      | 0.765
      | 0.7825
      | 0.8
      | ]
  Multiport Switch : MultiPortSwitch  Inputs=4  SaturateOnIntegerOverflow=off  InputSameDT=off
  Saturation : Saturate  UpperLimit=1000  LowerLimit=0
  NTractionControlKp : Outport  OutDataTypeStr=double  VectorParamsAs1DForOutWhenUnconnected=off
  wires:
  Gain3/1 -> Multiport Switch/5
  Gain2/1 -> Multiport Switch/4
  Gain1/1 -> Multiport Switch/3
  Multiport Switch/1 -> Saturation/1
  Kp1_linear_agg1/1 -> Gain1/1
  Kp1_linear_agg2/1 -> Gain2/1
  Kp1_linear_agg3/1 -> Gain3/1
  Kp1_linear_agg/1 -> Gain4/1
  NTractionControlKpSelector/1 -> Multiport Switch/1
  rSlipRatioError/1 -> Kp1_linear_agg/1, Kp1_linear_agg1/1, Kp1_linear_agg2/1, Kp1_linear_agg3/1
  Saturation/1 -> NTractionControlKp/1
  Gain4/1 -> Multiport Switch/2

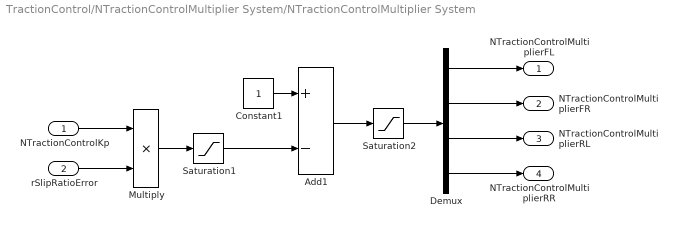
== system TractionControl/NTractionControlMultiplier System/NTractionControlMultiplier System ==
  NTractionControlKp : Inport  OutDataTypeStr=double
  rSlipRatioError : Inport  Port=2  OutDataTypeStr=double
  Add1 : Sum  Inputs=+-
  Constant1 : Constant
  Demux : Demux
  Multiply : Product
  Saturation1 : Saturate  UpperLimit=1  LowerLimit=0
  Saturation2 : Saturate  UpperLimit=1  LowerLimit=0
  NTractionControlMultiplierFL : Outport  OutDataTypeStr=double  VectorParamsAs1DForOutWhenUnconnected=off
  NTractionControlMultiplierFR : Outport  Port=2  OutDataTypeStr=double  VectorParamsAs1DForOutWhenUnconnected=off
  NTractionControlMultiplierRL : Outport  Port=3  OutDataTypeStr=double  VectorParamsAs1DForOutWhenUnconnected=off
  NTractionControlMultiplierRR : Outport  Port=4  OutDataTypeStr=double  VectorParamsAs1DForOutWhenUnconnected=off
  wires:
  Saturation1/1 -> Add1/2
  Add1/1 -> Saturation2/1
  Constant1/1 -> Add1/1
  rSlipRatioError/1 -> Multiply/2
  NTractionControlKp/1 -> Multiply/1
  Multiply/1 -> Saturation1/1
  Demux/1 -> NTractionControlMultiplierFL/1
  Demux/2 -> NTractionControlMultiplierFR/1
  Demux/4 -> NTractionControlMultiplierRR/1
  Demux/3 -> NTractionControlMultiplierRL/1
  Saturation2/1 -> Demux/1

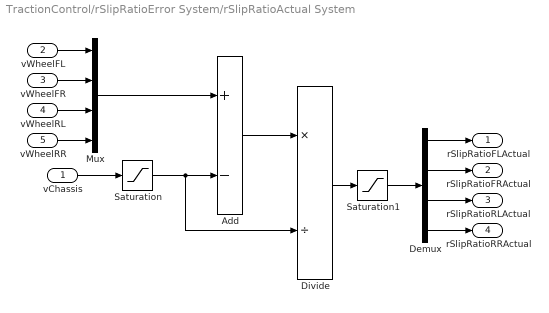
== system TractionControl/rSlipRatioError System/rSlipRatioActual System ==
  vChassis : Inport  OutDataTypeStr=double
  vWheelFL : Inport  Port=2  OutDataTypeStr=double  LockScale=on
  vWheelFR : Inport  Port=3  OutDataTypeStr=double  LockScale=on
  vWheelRL : Inport  Port=4  OutDataTypeStr=double  LockScale=on
  vWheelRR : Inport  Port=5  OutDataTypeStr=double  LockScale=on
  Add : Sum  Inputs=+-
  Demux : Demux
  Divide : Product  Inputs=*/
  Mux : Mux
  Saturation : Saturate  UpperLimit=50  LowerLimit=0.1
  Saturation1 : Saturate  UpperLimit=1000  LowerLimit=-1
  rSlipRatioFLActual : Outport  OutDataTypeStr=double  VectorParamsAs1DForOutWhenUnconnected=off
  rSlipRatioFRActual : Outport  Port=2  OutDataTypeStr=double  VectorParamsAs1DForOutWhenUnconnected=off
  rSlipRatioRLActual : Outport  Port=3  OutDataTypeStr=double  VectorParamsAs1DForOutWhenUnconnected=off
  rSlipRatioRRActual : Outport  Port=4  OutDataTypeStr=double  VectorParamsAs1DForOutWhenUnconnected=off
  wires:
  Mux/1 -> Add/1
  Saturation/1 -> Add/2, Divide/2
  vChassis/1 -> Saturation/1
  Divide/1 -> Saturation1/1
  Add/1 -> Divide/1
  vWheelRR/1 -> Mux/4
  vWheelRL/1 -> Mux/3
  vWheelFR/1 -> Mux/2
  vWheelFL/1 -> Mux/1
  Demux/4 -> rSlipRatioRRActual/1
  Demux/3 -> rSlipRatioRLActual/1
  Demux/2 -> rSlipRatioFRActual/1
  Demux/1 -> rSlipRatioFLActual/1
  Saturation1/1 -> Demux/1

== system TractionControl/rSlipRatioError System/rSlipRatioError System ==
  rSlipRatioOptimal : Inport  OutDataTypeStr=double
  rSlipRatioFLActual : Inport  Port=2  OutDataTypeStr=double
  rSlipRatioFRActual : Inport  Port=3  OutDataTypeStr=double
  rSlipRatioRLActual : Inport  Port=4  OutDataTypeStr=double
  rSlipRatioRRActual : Inport  Port=5  OutDataTypeStr=double
  Mux : Mux
  Subtract : Sum  Inputs=+-
  rSlipRatioError : Outport  OutDataTypeStr=double  VectorParamsAs1DForOutWhenUnconnected=off
  wires:
  Subtract/1 -> rSlipRatioError/1
  rSlipRatioOptimal/1 -> Subtract/2
  rSlipRatioFLActual/1 -> Mux/1
  rSlipRatioFRActual/1 -> Mux/2
  rSlipRatioRLActual/1 -> Mux/3
  rSlipRatioRRActual/1 -> Mux/4
  Mux/1 -> Subtract/1
